simulink model "H175_S3"  (R2023a)
settings: Solver=VariableStepAuto  StartTime=0.0  StopTime=1000  RelTol=1e-3
values from neighbouring files (symbols this model uses):
  Hydrowell_VTS =     [Hydrowell_values_VLV.mat]
undefined symbols (not defined in the file or in its folder): sigbuilder_block
libraries: fl_lib x107, nesl_utility x87, SimscapeFluids_lib x11, slpidlib x5
(part 1 of 8)
settings Model: Creator=adrian.taveras  LastModifiedBy=adrian.taveras

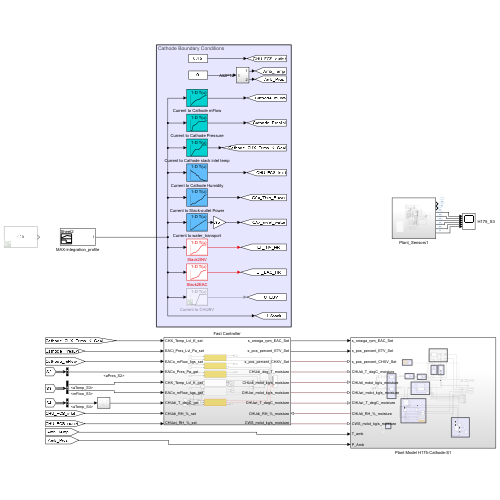
[thumbnail: Simulink's stored preview of the top-level diagram]
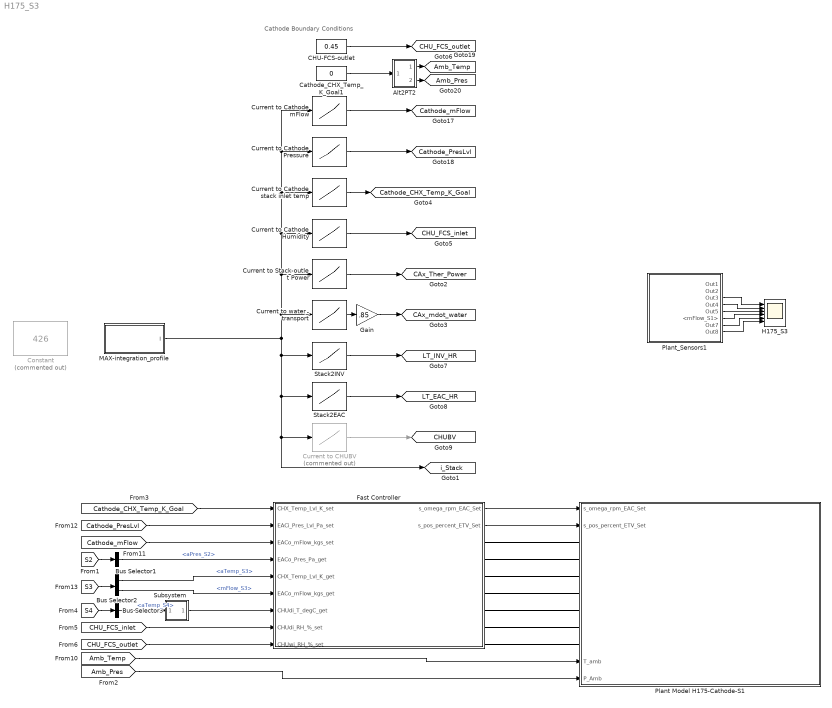
== system H175_S3 ==
  note: Cathode Boundary Conditions
  Alt2PT2 : Subsystem
  Bus Selector1 : BusSelector  OutputSignals=aPres_S2
  Bus Selector2 : BusSelector  OutputSignals=aTemp_S3,mFlow_S3
  Bus Selector3 : BusSelector  OutputSignals=aTemp_S4
  CHU-FCS-outlet : Constant  Value=0.45
  Cathode_CHX_Temp_K_Goal1 : Constant  Value=0
  Constant : Constant  Commented=on  Value=426
  Current to CHUBV : Lookup_n-D  Commented=on  NumberOfTableDimensions=1  BreakpointsForDimension1=[0;100;200;350;400;500;600]  Table=[0;0;0;1;1;1;1]  InternalRulePriority=Speed  RndMeth=Simplest
  Current to Cathode Humidity : Lookup_n-D  NumberOfTableDimensions=1  BreakpointsForDimension1=[20, 50, 100, 150, 200, 250, 300, 350, 400, 450, 500, 550, 600]  Table=[0.8,0.77,0.75,0.72,0.7,0.65,0.65,0.6,0.55,0.55,0.53,0.53,0.53]  InternalRulePriority=Speed  RndMeth=Simplest
  Current to Cathode Pressure : Lookup_n-D  NumberOfTableDimensions=1  BreakpointsForDimension1=[0;50;100;150;200;300;400;450;500;550;600]  Table=[112000;112000;170000;175000;180000;210000;210000;210000;210000;210000;230000]  InternalRulePriority=Speed  RndMeth=Simplest
  Current to Cathode mFlow : Lookup_n-D  NumberOfTableDimensions=1  BreakpointsForDimension1=[0;50;100;150;200;250;300;350;400;510;600]  Table=[0;0.03;0.05;0.07;0.0825;0.095;0.095;0.105;0.123;0.152;0.167]  InternalRulePriority=Speed  RndMeth=Simplest
  Current to Cathode stack inlet temp : Lookup_n-D  NumberOfTableDimensions=1  BreakpointsForDimension1=[20, 50, 100, 150, 200, 250, 300, 350, 400, 450, 500, 550, 600]  Table=[65,65,66,67,68,68,68,68,69,70,70,70,70]  InternalRulePriority=Speed  RndMeth=Simplest
  Current to Stack-outlet Power : Lookup_n-D  NumberOfTableDimensions=1  BreakpointsForDimension1=[20, 50, 100, 150, 200, 250, 300, 350, 400, 450, 500, 550, 600]  Table=[0.0274, 0.1198, 0.1925, 0.2134, 0.2502, 0.3358, 0.4478, 0.5224, 0.5988, 0.6756, 0.8257, 0.9909, 1.0339]*1000  InternalRulePriority=Speed  RndMeth=Simplest
  Current to water_transport : Lookup_n-D  NumberOfTableDimensions=1  BreakpointsForDimension1=[0;100;200;400;600]  Table=[0;4.247e-3;8.494e-3;1.697e-2;2.548e-2]  InternalRulePriority=Speed  RndMeth=Simplest
  Fast Controller : Subsystem
      settings: PortSchema="{\"entries\":[{\"content\":{\"sides\":[{\"content\":{\"connectorIds\":[\"Out1\",\"Out2\",\"LConn1\",\"LConn2\",\"LConn3\",\"LConn4\",\"LConn5\",\"LConn6\",\"LConn7\"]},\"type\":\"ConnectorPlacement.EquallySpacedRectSide\",\"uuid\":\"fec6d33c-3ad3-4174-acdc-3a3b9e5715f4\"},{\"content\":{\"connectorIds\":[\"In1\",\"In2\",\"In3\",\"In4\",\"In5\",\"In6\",\"In7\",\"In8\",\"In9\"],\"side\":\"RIGHT\"},\"type\":\"ConnectorPlacement.EquallySpacedRectSide\",\"uuid\":\"4aee90de-c0ab-447d-83f7-53a254285efe\"},{\"content\":{\"side\":\"TOP\"},\"type\":\"ConnectorPlacement.EquallySpacedRectSide\",\"uuid\":\"94b2adb1-5e3a-4413-84ea-fe1e13b8a59d\"}]},\"type\":\"ConnectorPlacement.EquallySpacedConnector\",\"uuid\":\"aca8449a-2e64-4d0b-80a0-10fe30b1ea20\"}],\"packageUris\":[\"http://schema.mathworks.com/mf0/Connector/R2020b\"],\"version\":\"1.0\"}"
  Gain : Gain  Gain=.85
  H175_S3 : Scope  NumInputPorts=6
  MAX-integration_profile : Subsystem  Tag=STV Subsys  LoadFcn=sigbuilder_block('load');  StartFcn=sigbuilder_block('start');  StopFcn=sigbuilder_block('stop');  ClipboardFcn=sigbuilder_block('clipboard');  mask(Sigbuilder block){tuvar=[0:10]}
      mask help: Simulink:masks:SigbuilderBlock_MD
      mask init:
      | if ~strcmp(get_param(bdroot(gcbh),'SimulationStatus'),'stopped') tuvar = sigbuilder_block('maskInit'); end
      settings: CopyFcn=sigbuilder_block('copy');  DeleteFcn=sigbuilder_block('delete');  ModelCloseFcn=sigbuilder_block('modelClose');  PreSaveFcn=sigbuilder_block('preSave');  PauseFcn=sigbuilder_block('pause');  ContinueFcn=sigbuilder_block('continue');  NameChangeFcn=sigbuilder_block('namechange');  OpenFcn=sigbuilder_block('open',[6 30.75 1428 715.5 ]);  CloseFcn=sigbuilder_block('close');
      mask Display: plot(0, 0, 100, 100,[2, 2, 32, 32, 2], [68, 8, 8, 68, 68],[32, 2], [38, 38], [32, 19, 2],[53, 60, 44], [32, 17, 17, 2],[16, 16, 31, 31]);txt = getActiveGroup(gcbh);text(2, 100, txt,'verticalAlignment', 'top');
  Plant Model H175-Cathode-S1 : Subsystem
      settings: PortSchema="{\"entries\":[{\"content\":{\"sides\":[{\"content\":{\"connectorIds\":[\"In1\",\"In2\",\"LConn1\",\"LConn2\",\"LConn3\",\"LConn4\",\"LConn5\",\"LConn6\",\"LConn7\",\"In3\",\"In4\"]},\"type\":\"ConnectorPlacement.EquallySpacedRectSide\",\"uuid\":\"e3b30cb5-20d3-4977-927f-9fea068a9234\"},{\"content\":{\"side\":\"RIGHT\"},\"type\":\"ConnectorPlacement.EquallySpacedRectSide\",\"uuid\":\"2d547627-9665-492a-afa4-fcc16b1173a1\"},{\"content\":{\"side\":\"TOP\"},\"type\":\"ConnectorPlacement.EquallySpacedRectSide\",\"uuid\":\"4ee6a80a-af1f-40b1-aa59-916ec7fe1294\"}]},\"type\":\"ConnectorPlacement.EquallySpacedConnector\",\"uuid\":\"0d82e4d1-cc18-4647-90fc-0df577891cdc\"}],\"packageUris\":[\"http://schema.mathworks.com/mf0/Connector/R2020b\"],\"version\":\"1.0\"}"
  Plant_Sensors1 : Subsystem
  Stack2EAC : Lookup_n-D  NumberOfTableDimensions=1  BreakpointsForDimension1=[0 100 200 300 400 500 600]  Table=[0;610;940;1760;3980;4620;5190]  InternalRulePriority=Speed  RndMeth=Simplest
  Stack2INV : Lookup_n-D  NumberOfTableDimensions=1  BreakpointsForDimension1=[0;100;200;300;400;500;600]  Table=[0;550;690;1450;2490;2870;2920]  InternalRulePriority=Speed  RndMeth=Simplest
  Subsystem : Subsystem
  tag scope: Amb_Pres=global, Amb_Temp=global, CAx_Ther_Power=global, CAx_mdot_water=global, CHUBV=global, CHU_FCS_inlet=global, CHU_FCS_outlet=global, Cathode_CHX_Temp_K_Goal=global, Cathode_PresLvl=global, Cathode_mFlow=global, LT_EAC_HR=global, LT_INV_HR=global, i_Stack=global
  wires:
  Plant_Sensors1/7(Out7) -> H175_S3/5
  Plant_Sensors1/8(Out8) -> H175_S3/6
  Plant_Sensors1/3(Out3) -> H175_S3/1
  Plant_Sensors1/6(<mFlow_S1>) -> H175_S3/4
  Plant_Sensors1/4(Out4) -> H175_S3/2
  Plant_Sensors1/5(Out5) -> H175_S3/3
  Current to Cathode stack inlet temp/1 -> [Cathode_CHX_Temp_K_Goal]
  Alt2PT2/2(Out2) -> [Amb_Pres]
  Current to Cathode mFlow/1 -> [Cathode_mFlow]
  Alt2PT2/1(Out1) -> [Amb_Temp]
  [CHU_FCS_inlet] -> Fast Controller/8(CHUdi_RH_%_set)
  Bus Selector3/1 -> Subsystem/1(<aTemp_S4>)  "<aTemp_S4>"
  [S2] -> Bus Selector1/1
  Fast Controller/1(s_omega_rpm_EAC_Set) -> Plant Model H175-Cathode-S1/1(s_omega_rpm_EAC_Set)
  Current to Cathode Pressure/1 -> [Cathode_PresLvl]
  Cathode_CHX_Temp_K_Goal1/1 -> Alt2PT2/1(In1)
  [CHU_FCS_outlet] -> Fast Controller/9(CHUwi_RH_%_set)
  [S4] -> Bus Selector3/1
  Fast Controller/2(s_pos_percent_ETV_Set) -> Plant Model H175-Cathode-S1/2(s_pos_percent_ETV_Set)
  CHU-FCS-outlet/1 -> [CHU_FCS_outlet]
  Subsystem/1(Out1) -> Fast Controller/7(CHUdi_T_degC_get)
  Bus Selector2/2 -> Fast Controller/6(EACo_mFlow_kgs_get)  "<mFlow_S3>"
  Bus Selector1/1 -> Fast Controller/4(EACo_Pres_Pa_get)  "<aPres_S2>"
  [Amb_Pres] -> Plant Model H175-Cathode-S1/4(P_Amb)
  [Cathode_CHX_Temp_K_Goal] -> Fast Controller/1(CHX_Temp_Lvl_K_set)
  Current to Cathode Humidity/1 -> [CHU_FCS_inlet]
  [S3] -> Bus Selector2/1
  [Cathode_PresLvl] -> Fast Controller/2(EACi_Pres_Lvl_Pa_set)
  [Cathode_mFlow] -> Fast Controller/3(EACo_mFlow_kgs_set)
  Bus Selector2/1 -> Fast Controller/5(CHX_Temp_Lvl_K_get)  "<aTemp_S3>"
  [Amb_Temp] -> Plant Model H175-Cathode-S1/3(T_amb)
  Current to Stack-outlet Power/1 -> [CAx_Ther_Power]
  Current to water_transport/1 -> Gain/1
  Gain/1 -> [CAx_mdot_water]
  MAX-integration_profile/1(I) -> Current to Cathode mFlow/1, Current to Cathode Pressure/1, Current to Cathode stack inlet temp/1, Current to Cathode Humidity/1, Current to Stack-outlet Power/1, Current to water_transport/1, Current to CHUBV/1, [i_Stack], Stack2EAC/1, Stack2INV/1
  Stack2INV/1 -> [LT_INV_HR]
  Stack2EAC/1 -> [LT_EAC_HR]
  Current to CHUBV/1 -> [CHUBV]
  connections:
  Plant Model H175-Cathode-S1/LConn3 -- Fast Controller/LConn3
  Plant Model H175-Cathode-S1/LConn1 -- Fast Controller/LConn1
  Plant Model H175-Cathode-S1/LConn2 -- Fast Controller/LConn2
  Plant Model H175-Cathode-S1/LConn5 -- Fast Controller/LConn5
  Plant Model H175-Cathode-S1/LConn6 -- Fast Controller/LConn6
  Plant Model H175-Cathode-S1/LConn7 -- Fast Controller/LConn7
  Plant Model H175-Cathode-S1/LConn4 -- Fast Controller/LConn4

== system H175_S3/Alt2PT2 ==
  In1 : Inport
  Add1 : Sum  Inputs=-+
  Constant4 : Constant  Value=0.0065
  Constant5 : Constant  Value=288.15
  Constant6 : Constant  Value=101330
  Constant7 : Constant  Value=4.256
  Constant8 : Constant  Value=288.15
  Divide1 : Product  Inputs=*/
  Math Function1 : Math  Operator=pow
  Product2 : Product
  Product3 : Product
  Out1 : Outport
  Out2 : Outport  Port=2
  wires:
  Constant5/1 -> Divide1/2
  Constant8/1 -> Add1/2
  In1/1 -> Product2/1
  Add1/1 -> Out1/1, Divide1/1
  Constant4/1 -> Product2/2
  Math Function1/1 -> Product3/1
  Constant7/1 -> Math Function1/2
  Divide1/1 -> Math Function1/1
  Product2/1 -> Add1/1
  Constant6/1 -> Product3/2
  Product3/1 -> Out2/1

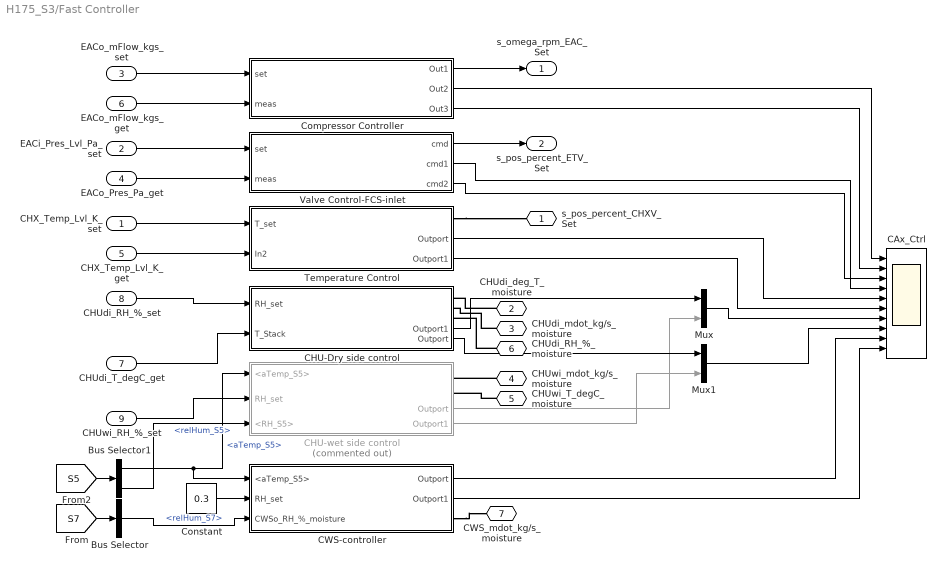
== system H175_S3/Fast Controller ==
  CHX_Temp_Lvl_K_set : Inport
  EACi_Pres_Lvl_Pa_set : Inport  Port=2
  EACo_mFlow_kgs_set : Inport  Port=3
  EACo_Pres_Pa_get : Inport  Port=4
  CHX_Temp_Lvl_K_get : Inport  Port=5
  EACo_mFlow_kgs_get : Inport  Port=6
  CHUdi_T_degC_get : Inport  Port=7
  CHUdi_RH_%_set : Inport  Port=8
  CHUwi_RH_%_set : Inport  Port=9
  Bus Selector : BusSelector  OutputSignals=relHum_S7
  Bus Selector1 : BusSelector  OutputSignals=aTemp_S5,relHum_S5
  CAx_Ctrl : Scope  NumInputPorts=10
  CHU-Dry side control : Subsystem
      settings: PortSchema="{\"entries\":[{\"content\":{\"sides\":[{\"content\":{\"connectorIds\":[\"In1\",\"In2\"]},\"type\":\"ConnectorPlacement.EquallySpacedRectSide\",\"uuid\":\"e04ad6f8-f772-4509-9e44-7e9617907586\"},{\"content\":{\"connectorIds\":[\"RConn1\",\"RConn2\",\"RConn3\",\"Out1\",\"Out2\"],\"side\":\"RIGHT\"},\"type\":\"ConnectorPlacement.EquallySpacedRectSide\",\"uuid\":\"0d864351-c193-45bf-90b1-984eb87a7782\"},{\"content\":{\"side\":\"TOP\"},\"type\":\"ConnectorPlacement.EquallySpacedRectSide\",\"uuid\":\"4c64baeb-8430-45ec-975f-7b4d4952dc8b\"}]},\"type\":\"ConnectorPlacement.EquallySpacedConnector\",\"uuid\":\"5dd74924-e120-426f-b6cd-4773f3c18ed2\"}],\"packageUris\":[\"http://schema.mathworks.com/mf0/Connector/R2020b\"],\"version\":\"1.0\"}"
  CHU-wet side control : Subsystem  Commented=on
      settings: PortSchema="{\"entries\":[{\"content\":{\"sides\":[{\"content\":{\"connectorIds\":[\"In1\",\"In2\",\"In3\"]},\"type\":\"ConnectorPlacement.EquallySpacedRectSide\",\"uuid\":\"5d784ad6-2694-4818-a8d0-e3f25f29943b\"},{\"content\":{\"connectorIds\":[\"RConn1\",\"RConn2\",\"Out1\",\"Out2\"],\"side\":\"RIGHT\"},\"type\":\"ConnectorPlacement.EquallySpacedRectSide\",\"uuid\":\"0f37eddd-db43-448e-bdba-1f3d3b9c7cf9\"},{\"content\":{\"side\":\"TOP\"},\"type\":\"ConnectorPlacement.EquallySpacedRectSide\",\"uuid\":\"2821bd82-ebdd-4ee5-8462-72507a5a1ef1\"}]},\"type\":\"ConnectorPlacement.EquallySpacedConnector\",\"uuid\":\"01309751-94c6-459a-9af4-24f452a07ce7\"}],\"packageUris\":[\"http://schema.mathworks.com/mf0/Connector/R2020b\"],\"version\":\"1.0\"}"
  CWS-controller : Subsystem
  "Compressor Controller " : Subsystem
  Constant : Constant  Value=0.3
  Mux : Mux  Inputs=2
  Mux1 : Mux  Inputs=2
  Temperature Control : Subsystem
      settings: PortSchema="{\"entries\":[{\"content\":{\"sides\":[{\"content\":{\"connectorIds\":[\"In1\",\"In2\"]},\"type\":\"ConnectorPlacement.EquallySpacedRectSide\",\"uuid\":\"e8458165-2262-49de-87f5-2c7bc958bbf7\"},{\"content\":{\"connectorIds\":[\"RConn1\",\"Out1\",\"Out2\"],\"side\":\"RIGHT\"},\"type\":\"ConnectorPlacement.EquallySpacedRectSide\",\"uuid\":\"42ad841b-551f-4f39-a141-2c874d3391ca\"},{\"content\":{\"side\":\"TOP\"},\"type\":\"ConnectorPlacement.EquallySpacedRectSide\",\"uuid\":\"fd6d4917-3fca-4949-93c2-24e90a6fe24c\"}]},\"type\":\"ConnectorPlacement.EquallySpacedConnector\",\"uuid\":\"b641fb00-fee4-4b18-b8cd-d00bddeb3481\"}],\"packageUris\":[\"http://schema.mathworks.com/mf0/Connector/R2020b\"],\"version\":\"1.0\"}"
  Valve Control-FCS-inlet : Subsystem
      settings: PortSchema="{\"entries\":[{\"content\":{\"sides\":[{\"content\":{\"connectorIds\":[\"Out1\",\"Out2\",\"Out3\"]},\"type\":\"ConnectorPlacement.EquallySpacedRectSide\",\"uuid\":\"8b9549d8-0479-4d9d-bb86-2520a85bd308\"},{\"content\":{\"connectorIds\":[\"In1\",\"In2\"],\"side\":\"RIGHT\"},\"type\":\"ConnectorPlacement.EquallySpacedRectSide\",\"uuid\":\"e3096e7f-7009-48fd-960b-05aa908ba84d\"},{\"content\":{\"side\":\"TOP\"},\"type\":\"ConnectorPlacement.EquallySpacedRectSide\",\"uuid\":\"4c3fd166-a148-4bd3-b47b-60debcc19f33\"}]},\"type\":\"ConnectorPlacement.EquallySpacedConnector\",\"uuid\":\"0022fa2c-fa81-4715-9695-0e1425952078\"}],\"packageUris\":[\"http://schema.mathworks.com/mf0/Connector/R2020b\"],\"version\":\"1.0\"}"
  s_pos_percent_CHXV_Set : PMIOPort  Side=Left
  CHUdi_deg_T_moisture : PMIOPort  Port=2  Side=Left
  CHUdi_mdot_kg/s_moisture : PMIOPort  Port=3  Side=Left
  CHUwi_mdot_kg/s_moisture : PMIOPort  Port=4  Side=Left
  CHUwi_T_degC_moisture : PMIOPort  Port=5  Side=Left
  CHUdi_RH_%_moisture : PMIOPort  Port=6  Side=Left
  CWS_mdot_kg/s_moisture : PMIOPort  Port=7  Side=Left
  s_omega_rpm_EAC_Set : Outport
  s_pos_percent_ETV_Set : Outport  Port=2
  wires:
  "Compressor Controller "/1(Out1) -> s_omega_rpm_EAC_Set/1
  CHX_Temp_Lvl_K_get/1 -> Temperature Control/2(In2)
  CHX_Temp_Lvl_K_set/1 -> Temperature Control/1(T_set)
  Valve Control-FCS-inlet/1(cmd) -> s_pos_percent_ETV_Set/1
  EACo_mFlow_kgs_get/1 -> "Compressor Controller "/2(meas)
  EACo_mFlow_kgs_set/1 -> "Compressor Controller "/1(set)
  EACi_Pres_Lvl_Pa_set/1 -> Valve Control-FCS-inlet/1(set)
  EACo_Pres_Pa_get/1 -> Valve Control-FCS-inlet/2(meas)
  "Compressor Controller "/2(Out2) -> CAx_Ctrl/1
  "Compressor Controller "/3(Out3) -> CAx_Ctrl/2
  Valve Control-FCS-inlet/2(cmd1) -> CAx_Ctrl/4
  Valve Control-FCS-inlet/3(cmd2) -> CAx_Ctrl/3
  CHUdi_T_degC_get/1 -> CHU-Dry side control/2(T_Stack)
  CHUdi_RH_%_set/1 -> CHU-Dry side control/1(RH_set)
  CHUwi_RH_%_set/1 -> CHU-wet side control/2(RH_set)
  Bus Selector/1 -> CWS-controller/3(CWSo_RH_%_moisture)  "<relHum_S7>"
  Constant/1 -> CWS-controller/2(RH_set)
  [S7] -> Bus Selector/1
  [S5] -> Bus Selector1/1
  Bus Selector1/1 -> CWS-controller/1(<aTemp_S5>), CHU-wet side control/1(<aTemp_S5>)  "<aTemp_S5>"
  Temperature Control/1(Outport) -> CAx_Ctrl/5
  Temperature Control/2(Outport1) -> CAx_Ctrl/6
  CHU-Dry side control/1(Outport1) -> Mux/1
  CHU-wet side control/1(Outport) -> Mux/2
  CHU-Dry side control/2(Outport) -> Mux1/1
  CHU-wet side control/2(Outport1) -> Mux1/2
  Mux/1 -> CAx_Ctrl/7
  Mux1/1 -> CAx_Ctrl/8
  CWS-controller/1(Outport) -> CAx_Ctrl/9
  CWS-controller/2(Outport1) -> CAx_Ctrl/10
  Bus Selector1/2 -> CHU-wet side control/3(<RH_S5>)  "<relHum_S5>"
  connections:
  Temperature Control/RConn1 -- s_pos_percent_CHXV_Set/RConn1
  CHUdi_deg_T_moisture/RConn1 -- CHU-Dry side control/RConn1
  CHUdi_mdot_kg/s_moisture/RConn1 -- CHU-Dry side control/RConn2
  CHUdi_RH_%_moisture/RConn1 -- CHU-Dry side control/RConn3
  CHUwi_mdot_kg/s_moisture/RConn1 -- CHU-wet side control/RConn1
  CHUwi_T_degC_moisture/RConn1 -- CHU-wet side control/RConn2
  CWS-controller/RConn1 -- CWS_mdot_kg/s_moisture/RConn1

== system H175_S3/MAX-integration_profile ==
  Demux : Demux  Tag=STV Demux  Outputs=1
      settings: DisplayOption=none
  FromWs : FromWorkspace  Tag=STV FromWs  VariableName=tuvar
      SigBuilderData=|
      | common.afterFinalStr = 'Extrapolate'
      | common.sampleTime = 0
      | dataSet.timeRange = [1 1000]
      | dataSet.name = 'Sheet2'
      | sbobj.Groups.Name = 'Sheet2'
      | sbobj.Groups.Signals.Name = 'I'
      | sbobj.Groups.Signals.XData = [1 200 220 400 420 600 620 800 820 1000]
      | sbobj.Groups.Signals.YData = [50 50 200 200 420 420 500 500 600 600]
      | sbobj.Groups.TimeRange = [1 16000]
  I : Outport  Tag=STV Outport
  wires:
  Demux/1 -> I/1
  FromWs/1 -> Demux/1
